simulink model "Symbol_Int"  (Simulink 7.4)
settings: Solver=ode45  StartTime=0.0  StopTime=0.01  RelTol=1e-3
values from neighbouring files (symbols this model uses):
  Ts = 0.000224*2176/9072/188    (= 2.85789335435e-07)    [Symbol_Int.m]
libraries: dspsnks4 x3, commblkintrlv2 x2, dspbuff3 x1, dspswit3 x1
settings Model: Creator=juan.gago  LastModifiedBy=juan.gago

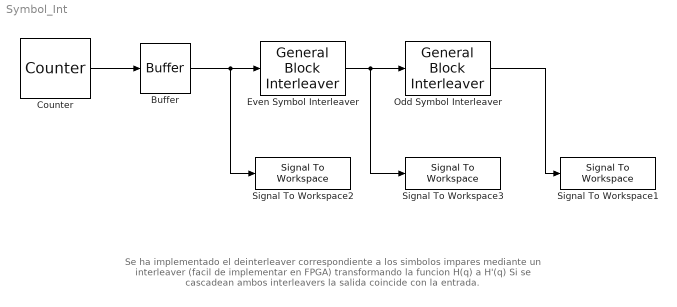
== system Symbol_Int ==
  note: Se ha implementado el deinterleaver correspondiente a los simbolos impares mediante un
      |  interleaver (facil de implementar en FPGA) transformando la funcion H(q) a H'(q)
      | Si se cascadean ambos interleavers la salida coincide con la entrada.
  Buffer : dspbuff3/Buffer  N=1512  V=0  ic=0
  Counter : dspswit3/Counter  Direction=Up  CountEvent=Free running  CounterSize=User defined  MaxCount=63  InitialCount=0  Output=Count  HitValue=32  ResetInput=off  SamplesPerFrame=1512  Ts=Ts  CntDtype=double  HitDtype=Logical
  Even Symbol Interleaver : commblkintrlv2/General Block Interleaver  elements=Hq_2k_pares
  Odd Symbol Interleaver : commblkintrlv2/General Block Interleaver  elements=Hq_2k_impares
  Signal To Workspace1 : dspsnks4/Signal To Workspace  SystemSampleTime=-1  VariableName=symbol_int  FrameMode=Concatenate frames (2-D array)
      settings: FixptAsFi=off
  Signal To Workspace2 : dspsnks4/Signal To Workspace  SystemSampleTime=-1  VariableName=bit_int  FrameMode=Concatenate frames (2-D array)
      settings: FixptAsFi=off
  Signal To Workspace3 : dspsnks4/Signal To Workspace  SystemSampleTime=-1  VariableName=intermedio  FrameMode=Concatenate frames (2-D array)
      settings: FixptAsFi=off
  wires:
  Counter/1 -> Buffer/1
  Buffer/1 -> Even Symbol Interleaver/1, Signal To Workspace2/1
  Odd Symbol Interleaver/1 -> Signal To Workspace1/1
  Even Symbol Interleaver/1 -> Signal To Workspace3/1, Odd Symbol Interleaver/1
